simulink model "AutoRS_Turm_Simulink"  (R2022b)
settings: Solver=FixedStepAuto  StartTime=0.0  StopTime=100  FixedStep=1e-4  RelTol=1e-3
settings Model: Creator=Sebastian  LastModifiedBy=Sebastian

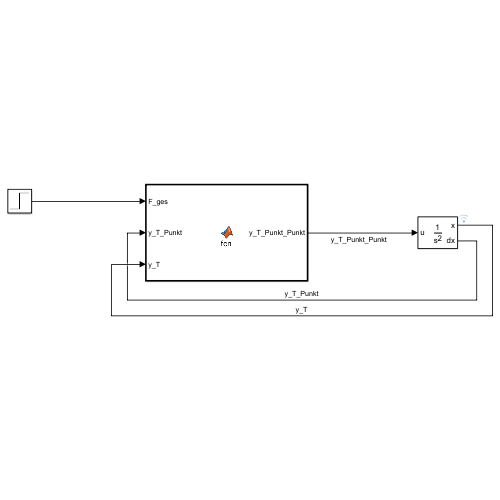
[thumbnail: Simulink's stored preview of the top-level diagram]
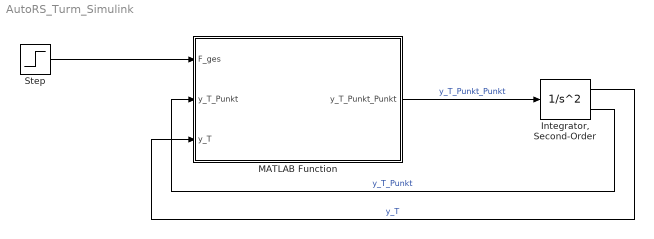
== system AutoRS_Turm_Simulink ==
  "Integrator, Second-Order" : SecondOrderIntegrator  ICX=0
  MATLAB Function : MATLAB Function  TreatAsAtomicUnit=on
  Step : Step  Time=0  After=1e7  SampleTime=0
  wires:
  MATLAB Function/1(y_T_Punkt_Punkt) -> "Integrator, Second-Order"/1  "y_T_Punkt_Punkt"
  "Integrator, Second-Order"/2 -> MATLAB Function/2(y_T_Punkt)  "y_T_Punkt"
  "Integrator, Second-Order"/1 -> MATLAB Function/3(y_T)  "y_T"
  Step/1 -> MATLAB Function/1(F_ges)

== matlab function AutoRS_Turm_Simulink/MATLAB Function ==
  data: F_ges input; y_T_Punkt input; y_T_Punkt_Punkt output; y_T input
function y_T_Punkt_Punkt = fcn(F_ges, y_T_Punkt, y_T)

    % KONSTANTEN
    c = Konstanten();
    
    % BERECHNUNG
    y_T_Punkt_Punkt = (F_ges-c.d_T*y_T_Punkt-c.k_T*y_T)/c.m_T;

end
